simulink model "mm_sim"  (R2025a)
settings: Solver=FixedStepAuto  StartTime=0.0  StopTime=10  RelTol=1e-3
libraries: mmuct_lib x2
settings Model: PacingRate=2  Creator=nicolls  LastModifiedBy=nicolls
settings RTWCC: GenCodeOnly=on

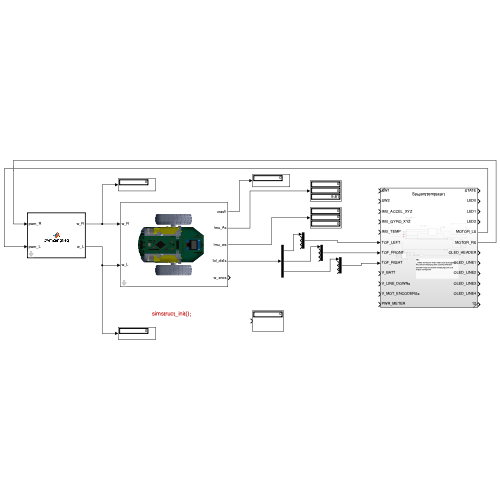
[thumbnail: Simulink's stored preview of the top-level diagram]
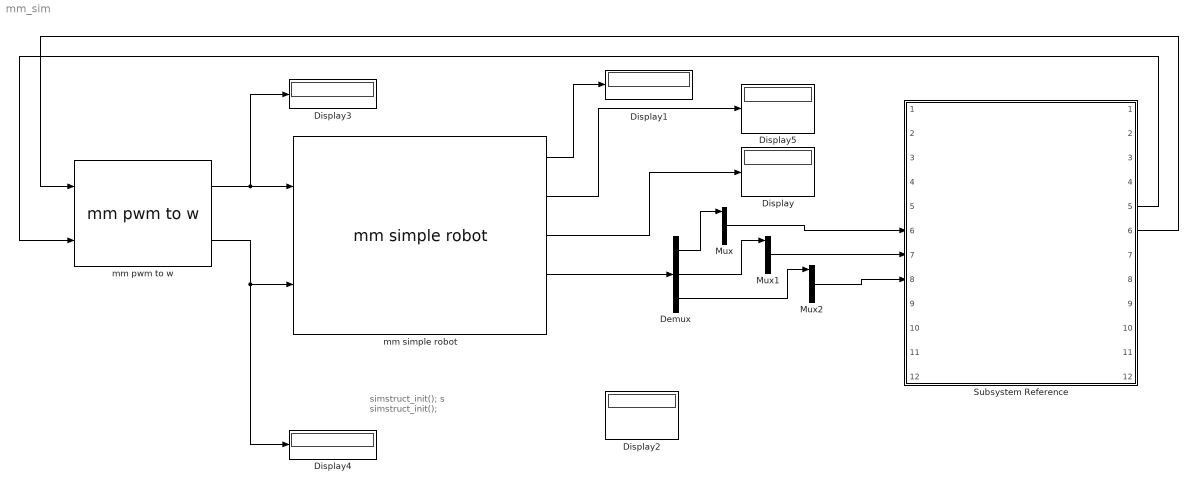
== system mm_sim ==
  note: simstruct_init();
      | s
      | simstruct_init();
  Demux : Demux  Outputs=3
  Display{,1..5} (6 alike) : Display
  Mux : Mux
  Mux1 : Mux
  Mux2 : Mux
  Subsystem Reference : Subsystem  ReferencedSubsystem=StudentTemplate1
  mm pwm to w : mmuct_lib/mm pwm to w  deadb=30  maxw=2*pi
  mm simple robot : mmuct_lib/mm simple robot  simstruct=simstruct  x0=0.1  y0=0.1  theta0=0
  wires:
  Demux/1 -> Mux/1
  Subsystem Reference/5 -> mm pwm to w/2
  Subsystem Reference/6 -> mm pwm to w/1
  Mux/1 -> Subsystem Reference/6
  Mux2/1 -> Subsystem Reference/8
  Mux1/1 -> Subsystem Reference/7
  Demux/2 -> Mux1/1
  Demux/3 -> Mux2/1
  mm pwm to w/2 -> Display4/1, mm simple robot/2
  mm pwm to w/1 -> mm simple robot/1, Display3/1
  mm simple robot/4 -> Demux/1
  mm simple robot/3 -> Display/1
  mm simple robot/2 -> Display5/1
  mm simple robot/1 -> Display1/1
